simulink model "Copy_of_simulator"  (R2024a)
settings: Solver=VariableStepAuto  StartTime=0.0  StopTime=50  RelTol=1e-3
values from neighbouring files (symbols this model uses):
  g = inputs(6,1)    [measFunction.m]    (also in stateFunction.m)
  k_f = 6.11e-8    (= 6.11e-08)    [Data.m]
  k_m = 1.5e-9    (= 1.5e-09)    [Data.m]
undefined symbols (not defined in the file or in its folder): A, B, C, L, m
libraries: slpidlib x7, simulink x2, shared6dof x1, sharedutil x1
(part 2 of 2)

== matlab function Copy_of_simulator/System_Dynamics/MATLAB Function ==
  data: ang input; o_R_b output
function o_R_b  = RotMatrix(ang)

phi = ang(1);
theta = ang(2);
psi = ang(3);

o_R_b = zeros(3,3);

% o_R_b = [cos(psi)*cos(theta),          ( -sin(psi)*cos(phi) -cos(psi)*sin(theta)*sin(phi) ),           ( sin(psi)*sin(phi) -cos(psi)*sin(theta)*cos(phi) );
%          sin(psi)*cos(theta),           ( cos(psi)*cos(phi) -sin(psi)*sin(theta)*sin(phi) ),          ( -cos(psi)*sin(phi) -sin(psi)*sin(theta)*cos(phi) );
%                   sin(theta),                                           cos(theta)*sin(phi),                                      cos(theta)*cos(phi)];

o_R_b = [cos(theta)*cos(psi),                                   cos(theta)*sin(psi),                                    -sin(theta);
         sin(phi)*sin(theta)*cos(psi) - cos(phi)*sin(psi),      sin(phi)*sin(theta)*sin(psi) + cos(phi)*cos(psi),       sin(phi)*cos(theta);
         cos(phi)*sin(theta)*cos(psi) + sin(phi)*sin(psi),      cos(phi)*sin(theta)*sin(psi) - sin(phi)*cos(psi),       cos(phi)*cos(theta)];
o_R_b = o_R_b';

end
